simulink model "pinn_degrade_v1"  (R2021b)
settings: Solver=ode4  StartTime=0.0  StopTime=test_length  FixedStep=step_size  RelTol=1e-3
values from neighbouring files (symbols this model uses):
  c = .2    (= 0.2)    [run_experiments_v1.m]
libraries: fl_lib x7, nesl_utility x5, sdl_lib x1
settings Model: Creator=dncob  LastModifiedBy=dncob

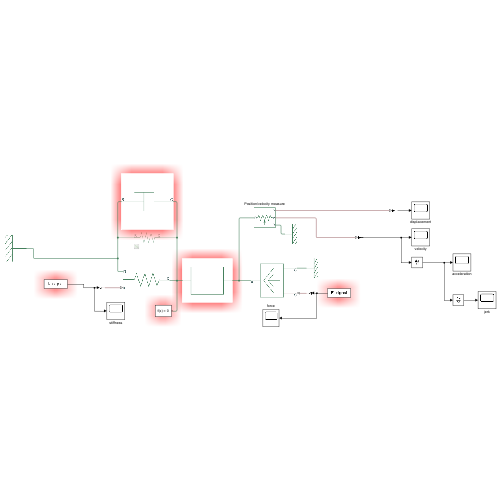
[thumbnail: Simulink's stored preview of the top-level diagram]
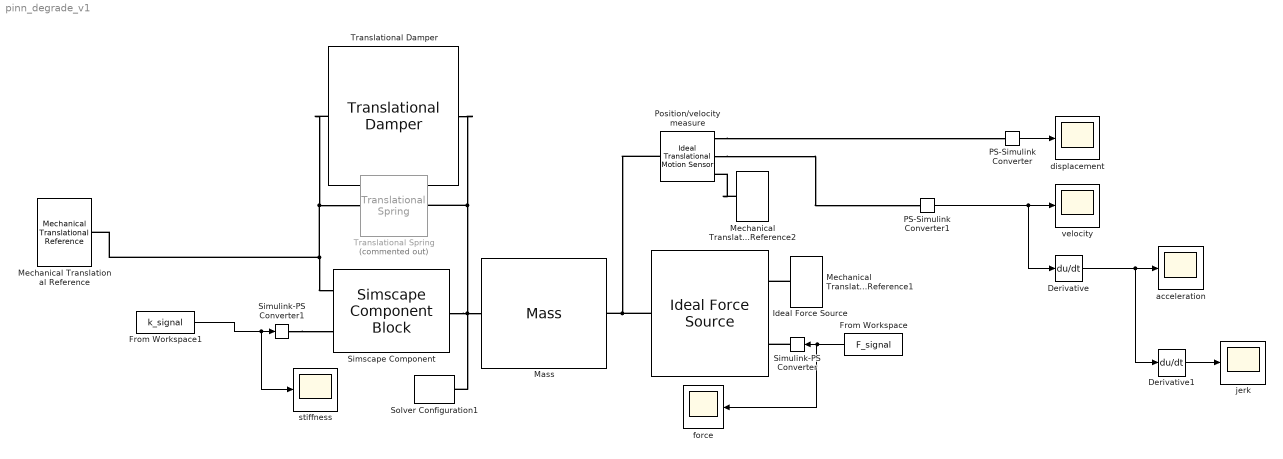
== system pinn_degrade_v1 ==
  Derivative : Derivative
  Derivative1 : Derivative
  From Workspace : FromWorkspace  VariableName=F_signal  SampleTime=-1  OutputAfterFinalValue=Holding final value
  From Workspace1 : FromWorkspace  VariableName=k_signal  SampleTime=-1  OutputAfterFinalValue=Holding final value
  Ideal Force Source : fl_lib/Mechanical/Mechanical Sources/Ideal Force Source
  Mass : fl_lib/Mechanical/Translational Elements/Mass  mass=m kg  num_ports=foundation.enum.numPorts2.two  v_specify=off  v_priority=High  v=0 m/s  v_nominal_specify=off  v_nominal_unit=m/s  v_nominal_value=1  f_specify=off  f_priority=None  f=0 N  f_nominal_specify=off  f_nominal_unit=N  f_nominal_value=1
      settings: InternalSimscapePortConfiguration="{\"Bottom\":[],\"Left\":[{\"id\":\"M\",\"label\":\"\",\"type\":\"foundation.mechanical.translational.translational\"}],\"Right\":[{\"id\":\"N\",\"label\":\"\",\"type\":\"foundation.mechanical.translational.translational\"}],\"Top\":[]}"
  Mechanical Translational Reference : fl_lib/Mechanical/Translational Elements/Mechanical Translational Reference
  Mechanical Translational Reference1 : fl_lib/Mechanical/Translational Elements/Mechanical Translational Reference
  Mechanical Translational Reference2 : fl_lib/Mechanical/Translational Elements/Mechanical Translational Reference
  PS-Simulink Converter : nesl_utility/PS-Simulink Converter  PhysicalDomain=network_engine_domain  SubClassName=ps_output  LeftPortType=input  RightPortType=output  PseudoPeriodic=off  Frequencies=[]  Unit=inherit  AffineConversion=off
      settings: SourceProductBaseCode=PW,SS
  PS-Simulink Converter1 : nesl_utility/PS-Simulink Converter  PhysicalDomain=network_engine_domain  SubClassName=ps_output  LeftPortType=input  RightPortType=output  PseudoPeriodic=off  Frequencies=[]  Unit=inherit  AffineConversion=off
      settings: SourceProductBaseCode=PW,SS
  Position/velocity measure : fl_lib/Mechanical/Mechanical Sensors/Ideal Translational Motion Sensor  offset=0 m
  Simscape Component : SimscapeComponentBlock  SourceFile=time_variable_spring  ComponentPath=time_variable_spring  ComponentVariants="[\"time_variable_spring\"]"  ComponentVariantNames="[\"time_variable_spring\"]"  ClassName=time_variable_spring  SchemaVersion=1  v_specify=off  v_priority=None  v=0 m/s  v_nominal_specify=off  v_nominal_unit=m/s  v_nominal_value=1  f_specify=off  f_priority=None  f=0 N  f_nominal_specify=off  f_nominal_unit=N  f_nominal_value=1  x_specify=off  x_priority=High  x=0 m  x_nominal_specify=off  x_nominal_unit=m  x_nominal_value=1
      settings: CopyFcn=simscape.engine.sli.internal.componentblockcallback(gcbh,'COPY')  PreCopyFcn=simscape.engine.sli.internal.componentblockcallback(gcbh,'PRECOPY')  PreDeleteFcn=simscape.engine.sli.internal.componentblockcallback(gcbh,'PREDELETE')  InternalSimscapePortConfiguration="{\"Bottom\":[],\"Left\":[{\"id\":\"R\",\"label\":\"R\",\"type\":\"foundation.mechanical.translational.translational\"},{\"id\":\"k\",\"label\":\"k\",\"type\":\"input\"}],\"Right\":[{\"id\":\"C\",\"label\":\"C\",\"type\":\"foundation.mechanical.translational.translational\"}],\"Top\":[]}"
      mask Type: Translational Spring
  Simulink-PS Converter : nesl_utility/Simulink-PS Converter  PhysicalDomain=network_engine_domain  SubClassName=ps_input  LeftPortType=input  RightPortType=output  PseudoPeriodic=off  Frequencies=[]  NoiseDistribution=none  NoiseParameters=[]  Unit=1  AffineConversion=off  FilteringAndDerivatives=provide  SimscapeFilterOrder=1  InputFilterTimeConstant=0.001  UdotUserProvided=0
      settings: SourceProductBaseCode=PW,SS
  Simulink-PS Converter1 : nesl_utility/Simulink-PS Converter  PhysicalDomain=network_engine_domain  SubClassName=ps_input  LeftPortType=input  RightPortType=output  PseudoPeriodic=off  Frequencies=[]  NoiseDistribution=none  NoiseParameters=[]  Unit=1  AffineConversion=off  FilteringAndDerivatives=provide  SimscapeFilterOrder=1  InputFilterTimeConstant=0.001  UdotUserProvided=0
      settings: SourceProductBaseCode=PW,SS
  Solver Configuration1 : nesl_utility/Solver Configuration  PhysicalDomain=network_engine_domain  SubClassName=solver  LeftPortType=input  RightPortType=generic  Tones=[]  Harmonics=[]  SimulateNoise=off  Profile=off  UseLocalSampling=off  EnableSwitchedLinearOptims=on  FrequencyDomain=off  UseCCode=off  RelTol=0.001  AbsTol=1e-06  MinStep=1e-09  ToWorkspace=off  RevertToSquareIcSolve=off  NumHomotopyIterations=100  PhasorMode=off  PhasorModeNumHarmonics=1  DoDC=off  ResidualTolerance=1e-09  UseLocalSolver=on  LocalSolverChoice=NE_TRAPEZOIDAL_ADVANCER  LocalSolverSampleTime=step_size  DoFixedCost=on  MaxNonlinIter=7  MaxModeIter=2  ComputeImpulses=off  ImpulseIterations=8  LinearAlgebra=Full  EquationFormulation=NE_TIME_EF  DelaysMemoryBudget=1024  AutomaticFiltering=on  FilteringTimeConstant=0.001  PartitionStorageMethod=AS_NEEDED  PartitionMemoryBudget=1024  PartitionMethod=FAST
      settings: SourceProductBaseCode=PW,SS
  Translational Damper : sdl_lib/Couplings & Drives/Springs & Dampers/Translational Damper  D=c N/(m/s)  enable_faults=simscape.enum.onoff.off  b_fault=1e6 N/(m/s)  temporal_fault=simscape.enum.onoff.off  fault_time=5 s  shock_fault=simscape.enum.onoff.off  acceleration_limit=100 m/s^2  shock_limit=1  report_fault=simscape.enum.assert.action.none  thermal_port=simscape.enum.thermaleffects.omit  thermal_mass=50 kJ/K  temperature_specify=off  temperature_priority=High  temperature=300 K  temperature_nominal_specify=off  temperature_nominal_unit=K  temperature_nominal_value=1
      settings: SourceProductBaseCode=LD
  Translational Spring : fl_lib/Mechanical/Translational Elements/Translational Spring  Commented=on  spr_rate=10 N/m  v_specify=off  v_priority=None  v=0 m/s  v_nominal_specify=off  v_nominal_unit=m/s  v_nominal_value=1  f_specify=off  f_priority=None  f=0 N  f_nominal_specify=off  f_nominal_unit=N  f_nominal_value=1  x_specify=off  x_priority=High  x=0 m  x_nominal_specify=off  x_nominal_unit=m  x_nominal_value=1
  acceleration : Scope
  displacement : Scope
  force : Scope
  jerk : Scope
  stiffness : Scope
  velocity : Scope
  wires:
  PS-Simulink Converter/1 -> displacement/1
  PS-Simulink Converter1/1 -> Derivative/1, velocity/1
  From Workspace/1 -> force/1, Simulink-PS Converter/1
  From Workspace1/1 -> stiffness/1, Simulink-PS Converter1/1
  Derivative/1 -> Derivative1/1, acceleration/1
  Derivative1/1 -> jerk/1
  connections:
  Ideal Force Source/LConn1 -- Position/velocity measure/LConn1 -- Mass/LConn1
  Simscape Component/RConn1 -- Translational Damper/RConn1 -- Translational Spring/RConn1 -- Mass/RConn1 -- Solver Configuration1/RConn1
  Position/velocity measure/RConn3 -- PS-Simulink Converter/LConn1
  Position/velocity measure/RConn2 -- PS-Simulink Converter1/LConn1
  Mechanical Translational Reference1/LConn1 -- Ideal Force Source/RConn2
  Simulink-PS Converter1/RConn1 -- Simscape Component/LConn2
  Simulink-PS Converter/RConn1 -- Ideal Force Source/RConn1
  Mechanical Translational Reference2/LConn1 -- Position/velocity measure/RConn1
  Simscape Component/LConn1 -- Translational Damper/LConn1 -- Translational Spring/LConn1 -- Mechanical Translational Reference/LConn1
